simulink model "Discr"  (R2023a)
settings: Solver=VariableStepAuto  StartTime=0.0  StopTime=10.0  RelTol=1e-3
values from neighbouring files (symbols this model uses):
  k = 5    [init.m]
  T1 = 0.4    [init.m]
  T2 = 0.05    [init.m]
settings Model: Creator=Алексей  LastModifiedBy=Алексей

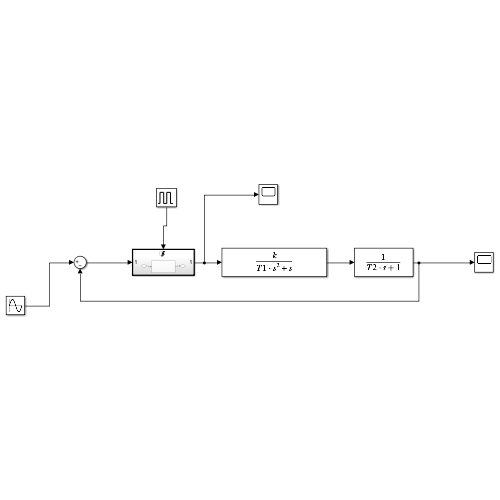
[thumbnail: Simulink's stored preview of the top-level diagram]
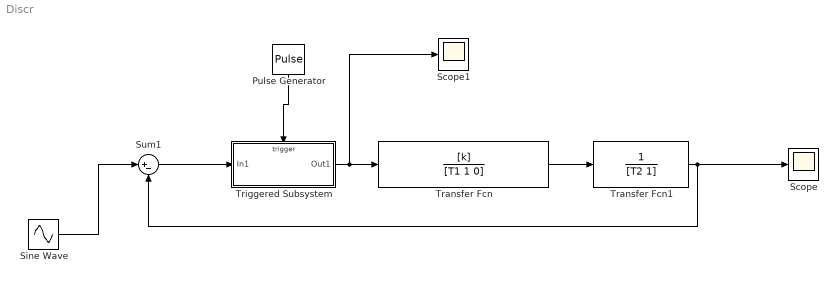
== system Discr ==
  Pulse Generator : DiscretePulseGenerator  PulseType=Time based  Period=0.01  PulseWidth=50
  Scope : Scope
  Scope1 : Scope
  Sine Wave : Sin  Amplitude=50  Frequency=0.5  SampleTime=0
  Sum1 : Sum  Inputs=|+-
  Transfer Fcn : TransferFcn  Numerator=[k]  Denominator=[T1 1 0]
  Transfer Fcn1 : TransferFcn  Denominator=[T2 1]
  Triggered Subsystem : Subsystem  TreatAsAtomicUnit=on
  wires:
  Transfer Fcn/1 -> Transfer Fcn1/1
  Transfer Fcn1/1 -> Scope/1, Sum1/2
  Sum1/1 -> Triggered Subsystem/1(In1)
  Triggered Subsystem/1(Out1) -> Scope1/1, Transfer Fcn/1
  Pulse Generator/1 -> Triggered Subsystem/Trigger
  Sine Wave/1 -> Sum1/1

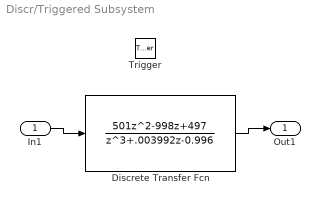
== system Discr/Triggered Subsystem ==
  In1 : Inport
  Trigger : TriggerPort  VariantControl=(inherit)
  Discrete Transfer Fcn : DiscreteTransferFcn  Numerator=[501 -998 497]  Denominator=[1 0 .003992 -0.996]
  Out1 : Outport
  wires:
  In1/1 -> Discrete Transfer Fcn/1
  Discrete Transfer Fcn/1 -> Out1/1
